simulink model "clock_input"  (R2021b)
settings: Solver=FixedStepAuto  StartTime=-9  StopTime=9  FixedStep=0.5  RelTol=1e-3
settings Model: Creator=Bhumil Depani  LastModifiedBy=Bhumil Depani
settings OptimizationCC: BlockReduction=off  DefaultParameterBehavior=Inlined  BufferReuse=off

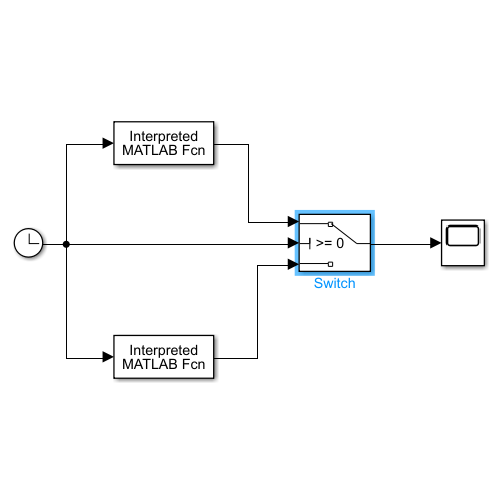
[thumbnail: Simulink's stored preview of the top-level diagram]
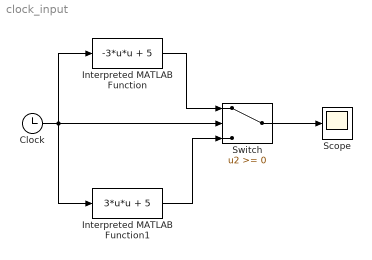
== system clock_input ==
  Clock : Clock
  Interpreted MATLAB Function : MATLABFcn  MATLABFcn=-3*u*u + 5  Output1D=off
  Interpreted MATLAB Function1 : MATLABFcn  MATLABFcn=3*u*u + 5
  Scope : Scope
  Switch : Switch
  wires:
  Clock/1 -> Interpreted MATLAB Function/1, Interpreted MATLAB Function1/1, Switch/2
  Interpreted MATLAB Function1/1 -> Switch/3
  Interpreted MATLAB Function/1 -> Switch/1
  Switch/1 -> Scope/1
